simulink model "downlink_4c2t"  (Simulink 8.7)
settings: Solver=VariableStepDiscrete  StartTime=0.0  StopTime=DUC_LINEUP_param.endTime  RelTol=1e-3
PreLoadFcn:
  | % Run the setup script when the model is opened
  | setup_downlink_4c2t;
InitFcn:
  | % Run the setup script again just before the
  | % model is run, so that any updates made
  | % after opening are applied.
  | setup_downlink_4c2t;
  | 
  | %% DSPBuilder Start
  | alt_dspbuilder_update_model(bdroot)
  | %% DSPBuilder End
values from neighbouring files (symbols this model uses):
  LUTS_DPD_CLIP =     [downlink_4c2t_dpd_clip.mat]
  PulsExtention = 128    [setup_downlink_4c2t.m]
  StartAddress1 = Iter1_Param.BaseAddr + 3200    [setup_downlink_4c2t.m]
  StartAddress2 = StartAddress1+1024    [setup_downlink_4c2t.m]
  win = [w(1:PulsExtention) ones(1,Iter0_Param.pulseLen) w(PulsExtention+1:end)]    [setup_downlink_4c2t.m]
undefined symbols (not defined in the file or in its folder): AdvDSPBChannelOutDisplay, AdvDSPBDMemDisplay, dpoly, dspba_ChannelInVis, dspba_ChannelOutVis, dspba_internal_get_channel_ports, dspba_internal_get_demux_ports, DUC_LINEUP_param, evalAionMaskParam, iq_width, Iter0_Param, latency, primtype, REG, UseDontCare, value
undefined symbols (not defined in the file): cfr0_id, cfr_Params0, cfr_Params1, clock_rate, REG_dut_id_addr
libraries: DSPBAPrim x1438, DSPBAControl x77, DSPBAModelBus x71, DSPBABase x40, downlink_4c2t_foldingcfr_3firs_lib x26, DSPBAUtilities x8, downlink_4c2t_lib x4, downlink_4c2t_cordic_lib x2, downlink_4c2t_dpd_clipper x2, DSPBAFilters x2, DSPBAWaveformSynth x2, downlink_4c2t_lduc_lib x1
(part 3 of 17)

== system downlink_4c2t/DUT/Gain_duc_input ==
  a : Inport
  v : Inport  Port=2
  c : Inport  Port=3
  carr1_gain_val : Inport  Port=4
  carr2_gain_val : Inport  Port=5
  carr3_gain_val : Inport  Port=6
  carr4_gain_val : Inport  Port=7
  carr5_gain_val : Inport  Port=8
  carr6_gain_val : Inport  Port=9
  carr7_gain_val : Inport  Port=10
  carr8_gain_val : Inport  Port=11
  Term : Terminator
  gain : Subsystem
  scale_gain : DSPBABase/Scale  otype=sfix(16 )  scale=2^-15  rndmethod=Unbiased  factor=1  satmethod=Symmetric  shift_vec=0  latency=7  wideSimulation=off  version=20090407
  zero_idx : DSPBAPrim/Const  primtype=const  nInputs=0  nOutputs=1  omode=Inherit via internal rule  otype=sfix(16)  scale=2^-15  rndmethod=Unbiased  factor=1  satmethod=Symmetric  shift_vec=[0 1 2 -1]  value=0  inPortNames=['+'; '+';]  outPortNames=[' ']  dspbaimage=dspba_prim.jpg  text=fprintf('%s', num2str(value));  style=Optimised  visibilities=8 + 1024  floatPrecision=float32_m23  version=20120820
  gain_v_out : Outport
  gain_c_out : Outport  Port=2
  gain_real_out : Outport  Port=3
  wires:
  a/1 -> gain/1(a)
  v/1 -> gain/2(v)
  c/1 -> gain/3(c)
  scale_gain/4 -> Term/1
  zero_idx/1 -> scale_gain/4
  gain/1(gain_v_out) -> scale_gain/2
  gain/2(gain_c_out) -> scale_gain/3
  gain/3(gain_real_out) -> scale_gain/1
  scale_gain/1 -> gain_real_out/1
  scale_gain/2 -> gain_v_out/1
  scale_gain/3 -> gain_c_out/1
  carr1_gain_val/1 -> gain/4(carr1_gain_val)
  carr2_gain_val/1 -> gain/5(carr2_gain_val)
  carr3_gain_val/1 -> gain/6(carr3_gain_val)
  carr4_gain_val/1 -> gain/7(carr4_gain_val)
  carr5_gain_val/1 -> gain/8(carr5_gain_val)
  carr6_gain_val/1 -> gain/9(carr6_gain_val)
  carr7_gain_val/1 -> gain/10(carr7_gain_val)
  carr8_gain_val/1 -> gain/11(carr8_gain_val)

== system downlink_4c2t/DUT/Gain_summer ==
  a : Inport
  v : Inport  Port=2
  c : Inport  Port=3
  Ant1_gain_val : Inport  Port=4
  Antr2_gain_val : Inport  Port=5
  Subsystem : Subsystem
  Term : Terminator
  scale_gain : DSPBABase/Scale  otype=sfix(16 )  scale=2^-15  rndmethod=Unbiased  factor=1  satmethod=Symmetric  shift_vec=0  latency=7  wideSimulation=off  version=20090407
  zero_idx : DSPBAPrim/Const  primtype=const  nInputs=0  nOutputs=1  omode=Inherit via internal rule  otype=sfix(16)  scale=2^-15  rndmethod=Unbiased  factor=1  satmethod=Symmetric  shift_vec=[0 1 2 -1]  value=0  inPortNames=['+'; '+';]  outPortNames=[' ']  dspbaimage=dspba_prim.jpg  text=fprintf('%s', num2str(value));  style=Optimised  visibilities=8 + 1024  floatPrecision=float32_m23  version=20120820
  gain_real_out : Outport
  gain_v_out : Outport  Port=2
  gain_c_out : Outport  Port=3
  wires:
  Antr2_gain_val/1 -> Subsystem/5(ant2_gain_val)
  Ant1_gain_val/1 -> Subsystem/4(ant1_gain_val)
  scale_gain/3 -> gain_c_out/1
  scale_gain/2 -> gain_v_out/1
  scale_gain/1 -> gain_real_out/1
  Subsystem/3(gain_real_out) -> scale_gain/1
  Subsystem/2(gain_c_out) -> scale_gain/3
  Subsystem/1(gain_v_out) -> scale_gain/2
  zero_idx/1 -> scale_gain/4
  scale_gain/4 -> Term/1
  c/1 -> Subsystem/3(c)
  v/1 -> Subsystem/2(v)
  a/1 -> Subsystem/1(a)

== system downlink_4c2t/DUT/HDUC_STG1 ==
  a1 : Inport
  v : Inport  Port=2
  c : Inport  Port=3
  Const5 : DSPBAPrim/Const  primtype=const  nInputs=0  nOutputs=1  omode=Inherit via internal rule  otype=sfix(16)  scale=2^-15  rndmethod=Unbiased  factor=1  satmethod=Symmetric  shift_vec=[0 1 2 -1]  value=0  inPortNames=['+'; '+';]  outPortNames=[' ']  dspbaimage=dspba_prim.jpg  text=fprintf('%s', num2str(value));  style=Optimised  visibilities=8 + 1024  floatPrecision=float32_m23  version=20120820
  HB_filter6 : DSPBAFilters/InterpolatingFIR  nInputRate=DUC_LINEUP_param.HB_filt6.SampleRate  interp=DUC_LINEUP_param.HB_filt6.Interpolation  nchan=DUC_LINEUP_param.HB_filt6.ChanCount  symmetry=Symmetrical  coef=DUC_LINEUP_param.HB_filt6.coeffs(1,:)  addr=DUC_LINEUP_param.HB_filt6.base_addr1  rwmode=Read/Write  nband=Half Band  exposebus=off  latency=9  version=20090407  recon=off  MM=[0,1,2,3,4,5,6,7,8,9,10,11,12,13,14,15]
  Terminator : Terminator
  scale_HB_filter6 : DSPBABase/Scale  otype=sfix(DUC_LINEUP_param.output_word_length)  scale=2^-DUC_LINEUP_param.output_fraction_length  rndmethod=Truncate  factor=[1 1]  satmethod=Symmetric  shift_vec=[1 1]  latency=7  wideSimulation=off  version=20090407
  q1 : Outport
  qv : Outport  Port=2
  qc : Outport  Port=3
  wires:
  scale_HB_filter6/1 -> q1/1
  scale_HB_filter6/3 -> qc/1
  HB_filter6/3 -> scale_HB_filter6/3
  HB_filter6/2 -> scale_HB_filter6/2
  scale_HB_filter6/2 -> qv/1
  HB_filter6/1 -> scale_HB_filter6/1
  Const5/1 -> scale_HB_filter6/4
  v/1 -> HB_filter6/2
  c/1 -> HB_filter6/3
  a1/1 -> HB_filter6/1
  scale_HB_filter6/4 -> Terminator/1

== system downlink_4c2t/DUT/HDUC_STG2 ==
  a1 : Inport
  v : Inport  Port=2
  c : Inport  Port=3
  Const5 : DSPBAPrim/Const  primtype=const  nInputs=0  nOutputs=1  omode=Specify via dialog  otype=ufix(2)  scale=2^-0  rndmethod=Unbiased  factor=1  satmethod=Symmetric  shift_vec=[0 1 2 -1]  value=0  inPortNames=['+'; '+';]  outPortNames=[' ']  dspbaimage=dspba_prim.jpg  text=fprintf('%s', num2str(value));  style=Optimised  visibilities=8 + 1024  floatPrecision=float32_m23  version=20120820
  HB_filter7 : DSPBAFilters/InterpolatingFIR  nInputRate=DUC_LINEUP_param.HB_filt7.SampleRate  interp=DUC_LINEUP_param.HB_filt7.Interpolation  nchan=DUC_LINEUP_param.HB_filt7.ChanCount  symmetry=Symmetrical  coef=DUC_LINEUP_param.HB_filt7.coeffs(1,:)  addr=DUC_LINEUP_param.HB_filt7.base_addr1  rwmode=Read/Write  nband=Half Band  exposebus=off  latency=7  version=20090407  recon=off  MM=[0,1,2,3,4,5,6,7,8,9,10,11,12,13,14,15]
  Terminator : Terminator
  scale_HB_filter6 : DSPBABase/Scale  otype=sfix(DUC_LINEUP_param.output_word_length)  scale=2^-DUC_LINEUP_param.output_fraction_length  rndmethod=Truncate  factor=[1 1 1 1]  satmethod=Symmetric  shift_vec=[1 1 1 1]  latency=7  wideSimulation=off  version=20090407
  q1 : Outport
  qv : Outport  Port=2
  qc : Outport  Port=3
  wires:
  scale_HB_filter6/1 -> q1/1
  scale_HB_filter6/3 -> qc/1
  HB_filter7/3 -> scale_HB_filter6/3
  HB_filter7/2 -> scale_HB_filter6/2
  scale_HB_filter6/2 -> qv/1
  HB_filter7/1 -> scale_HB_filter6/1
  Const5/1 -> scale_HB_filter6/4
  v/1 -> HB_filter7/2
  c/1 -> HB_filter7/3
  a1/1 -> HB_filter7/1
  scale_HB_filter6/4 -> Terminator/1

== system downlink_4c2t/DUT/LDUC ==
  In_v : Inport
  In_c : Inport  Port=2
  In_d : Inport  Port=3
  In_sync_pulse : Inport  Port=4
  sum_shift : Inport  Port=5
  LDUC : downlink_4c2t_lduc_lib/LDUC1  clock_margin=DUC_LINEUP_param.ClockMargin_DUC  chan_filter_base_addr=DUC_LINEUP_param.chan_filter.base_addr1  hb4_base_addr=DUC_LINEUP_param.HB_filt4.base_addr1  hb5_base_addr=DUC_LINEUP_param.HB_filt5.base_addr1  hb5_2_base_addr=DUC_LINEUP_param.HB_filt5_2.base_addr1
      link override Channal_Filter/SingleRateFIR: latency=4
      link override Channal_Filter/scale_HB_filter1: latency=4
      link override HB4/HB4/HB_filter4: latency=15
      link override HB4/HB4/scale_HB_filter4: latency=4
      link override HB5/HB_filter5: latency=11
      link override HB5/HB_filter_2: latency=11
      link override HB5/PipeReg1/ChannelOut: value=1  packetBeginEnabled=off  latency=1
      link override HB5/PipeReg2/ChannelOut: value=1  packetBeginEnabled=off  latency=1
      link override HB5/PipeReg3/ChannelOut: value=1  packetBeginEnabled=off  latency=1
      link override HB5/PipeReg4/ChannelOut: value=1  packetBeginEnabled=off  latency=1
      link override HB5/scale_HB_filter5: latency=4
      link override PipeReg/ChannelOut: value=1  packetBeginEnabled=off  latency=2
      link override PipeReg1/ChannelOut: value=1  packetBeginEnabled=off  latency=1
      link override PipeReg2/ChannelOut: value=1  packetBeginEnabled=off  latency=2
      link override PipeReg3/ChannelOut: value=1  packetBeginEnabled=off  latency=1
      link override PipeReg4/ChannelOut: value=1  packetBeginEnabled=off  latency=2
      link override PipeReg5/ChannelOut: value=1  packetBeginEnabled=off  latency=2
  Mixer_Summer : Subsystem
  PipeReg_avln_lduc_L : downlink_4c2t_foldingcfr_3firs_lib/PipeReg  NPipe=2  Clock_Margin=DUC_LINEUP_param.ClockMargin
      link override ChannelOut: latency=2  value=1  packetBeginEnabled=off
  PipeReg_avln_lduc_R : downlink_4c2t_foldingcfr_3firs_lib/PipeReg  NPipe=2  Clock_Margin=DUC_LINEUP_param.ClockMargin
      link override ChannelOut: latency=2  value=1  packetBeginEnabled=off
  Out1 : Outport
  Out2 : Outport  Port=2
  Out3 : Outport  Port=3
  wires:
  PipeReg_avln_lduc_R/1 -> LDUC/1
  PipeReg_avln_lduc_R/2 -> LDUC/2
  In_v/1 -> PipeReg_avln_lduc_L/2
  In_d/1 -> PipeReg_avln_lduc_L/1
  PipeReg_avln_lduc_L/2 -> PipeReg_avln_lduc_R/2
  PipeReg_avln_lduc_L/3 -> PipeReg_avln_lduc_R/3
  In_c/1 -> PipeReg_avln_lduc_L/3
  PipeReg_avln_lduc_R/3 -> LDUC/3
  In_sync_pulse/1 -> Mixer_Summer/4(In_sync_pulse)
  LDUC/1 -> Mixer_Summer/1(In_a)
  LDUC/2 -> Mixer_Summer/2(In_V)
  LDUC/3 -> Mixer_Summer/3(In_C)
  Mixer_Summer/3(Out_C) -> Out3/1
  Mixer_Summer/1(Out_q) -> Out1/1
  Mixer_Summer/2(Out_V) -> Out2/1
  PipeReg_avln_lduc_L/1 -> PipeReg_avln_lduc_R/1
  sum_shift/1 -> Mixer_Summer/5(sum_shift)

== system downlink_4c2t/DUT/REAL_COMPLEX1 ==
  a1 : Inport
  v : Inport  Port=2
  c : Inport  Port=3
  ChannelIn : DSPBAPrim/ChannelIn  primtype=channelin  nInputs=dspba_internal_get_channel_ports(gcb)  nOutputs=dspba_internal_get_channel_ports(gcb)  omode=Inherit via internal rule  otype=sfix(16)  scale=2^-15  rndmethod=Unbiased  factor=1  satmethod=Symmetric  shift_vec=[0 1 2 -1]  value=1  inPortNames=['v'; 'c'; '0'; '1'; '2'; '3'; '4'; '5'; '6'; '7'; '8'; '9'; 'A'; 'B'; 'D'; 'E'; 'F'; 'G'; 'H'; 'I'; 'J'; 'K'; 'L'; 'M'; 'N'; 'O'; 'P'; 'Q'; 'R'; 'S'; 'T'; 'U'; 'W'; 'X'; 'Y'; 'Z']  outPortNames=['v'; 'c'; '0'; '1'; '2'; '3'; '4'; '5'; '6'; '7'; '8'; '9'; 'A'; 'B'; 'D'; 'E'; 'F'; 'G'; 'H'; 'I'; 'J'; 'K'; 'L'; 'M'; 'N'; 'O'; 'P'; 'Q'; 'R'; 'S'; 'T'; 'U'; 'W'; 'X'; 'Y'; 'Z']  dspbaimage=dspba_prim.jpg  text=fprintf('In');  style=Optimised  dataSignals=1  foldingEnabled=off  channels=1  sampleRate=200  packetBeginPresent=off  packetBeginEnabled=off  visibilities=dspba_ChannelInVis(gcb)  latencyCorrection=0  version=20141013
  ChannelOut : DSPBAPrim/ChannelOut  primtype=channelout  nInputs=dspba_internal_get_channel_ports(gcb)  nOutputs=dspba_internal_get_channel_ports(gcb)  omode=Inherit via internal rule  otype=sfix(16)  scale=2^-15  rndmethod=Unbiased  factor=1  satmethod=Symmetric  shift_vec=[0 1 2 -1]  value=4  inPortNames=['v'; 'c'; '0'; '1'; '2'; '3'; '4'; '5'; '6'; '7'; '8'; '9'; 'A'; 'B'; 'D'; 'E'; 'F'; 'G'; 'H'; 'I'; 'J'; 'K'; 'L'; 'M'; 'N'; 'O'; 'P'; 'Q'; 'R'; 'S'; 'T'; 'U'; 'W'; 'X'; 'Y'; 'Z']  outPortNames=['v'; 'c'; '0'; '1'; '2'; '3'; '4'; '5'; '6'; '7'; '8'; '9'; 'A'; 'B'; 'D'; 'E'; 'F'; 'G'; 'H'; 'I'; 'J'; 'K'; 'L'; 'M'; 'N'; 'O'; 'P'; 'Q'; 'R'; 'S'; 'T'; 'U'; 'W'; 'X'; 'Y'; 'Z']  dspbaimage=dspba_prim.jpg  text=fprintf('Out%s', AdvDSPBChannelOutDisplay(latency));  style=Optimised  dataSignals=4  foldingEnabled=off  channels=1  sampleRate=200  packetBeginPresent=off  packetBeginEnabled=off  visibilities=dspba_ChannelOutVis(gcb)  latency=0  latencyCorrection=0  version=20141013
  Const : DSPBAPrim/Const  primtype=const  nInputs=0  nOutputs=1  omode=Inherit via internal rule  otype=sfix(16)  scale=2^-15  rndmethod=Unbiased  factor=1  satmethod=Symmetric  shift_vec=[0 1 2 -1]  value=0  inPortNames=['+'; '+';]  outPortNames=[' ']  dspbaimage=dspba_prim.jpg  text=fprintf('%s', num2str(value));  style=Optimised  visibilities=8 + 1024  floatPrecision=float32_m23  version=20120820
  Demux4 : Demux
  LocalThreshold : DSPBABase/LocalThreshold  margin=DUC_LINEUP_param.ClockMargin  delayRegOrRAMThresholdBits=-1  MediumDualMemThresholdBits=-1  LargeDualMemThresholdBits=-1  hardMultiplierThresholdLuts=-1  complexMultKaratsuba=off  version=0
  Real-Imag to Complex : RealImagToComplex
  Real-Imag to Complex1 : RealImagToComplex
  SynthesisInfo : DSPBAPrim/SynthesisInfo  primtype=synthinfo  nInputs=0  nOutputs=0  omode=Inherit via internal rule  otype=sfix(16)  scale=2^-15  rndmethod=Truncate  factor=1  satmethod=Symmetric  shift_vec=[0 1 2 -1]  value=99  inPortNames=[' '; ' ';]  outPortNames=[' ']  dspbaimage=dspba_prim_ctrl.jpg  text=fprintf('Style=%s', style);  style=Scheduled  visibilities=2^15+2^17+2^18+2^19  constraintInUse=off  constraintRelation=>  constraintLimit=20  bitAccurate=off  version=20150220
  Terminator17 : Terminator
  q1 : Outport
  q2 : Outport  Port=2
  q_v : Outport  Port=3
  q_c : Outport  Port=4
  wires:
  ChannelOut/3 -> Real-Imag to Complex/1
  Demux4/2 -> ChannelOut/4
  Demux4/4 -> ChannelOut/6
  Demux4/3 -> ChannelOut/5
  ChannelIn/2 -> Terminator17/1
  Const/1 -> ChannelOut/2
  ChannelIn/1 -> ChannelOut/1
  Demux4/1 -> ChannelOut/3
  ChannelIn/3 -> Demux4/1
  Real-Imag to Complex/1 -> q1/1
  ChannelOut/4 -> Real-Imag to Complex/2
  ChannelOut/2 -> q_c/1
  ChannelOut/1 -> q_v/1
  c/1 -> ChannelIn/2
  v/1 -> ChannelIn/1
  a1/1 -> ChannelIn/3
  Real-Imag to Complex1/1 -> q2/1
  ChannelOut/5 -> Real-Imag to Complex1/1
  ChannelOut/6 -> Real-Imag to Complex1/2

== system downlink_4c2t/DUT/REAL_COMPLEX2 ==
  a1 : Inport
  v : Inport  Port=2
  c : Inport  Port=3
  ChannelIn : DSPBAPrim/ChannelIn  primtype=channelin  nInputs=dspba_internal_get_channel_ports(gcb)  nOutputs=dspba_internal_get_channel_ports(gcb)  omode=Inherit via internal rule  otype=sfix(16)  scale=2^-15  rndmethod=Unbiased  factor=1  satmethod=Symmetric  shift_vec=[0 1 2 -1]  value=1  inPortNames=['v'; 'c'; '0'; '1'; '2'; '3'; '4'; '5'; '6'; '7'; '8'; '9'; 'A'; 'B'; 'D'; 'E'; 'F'; 'G'; 'H'; 'I'; 'J'; 'K'; 'L'; 'M'; 'N'; 'O'; 'P'; 'Q'; 'R'; 'S'; 'T'; 'U'; 'W'; 'X'; 'Y'; 'Z']  outPortNames=['v'; 'c'; '0'; '1'; '2'; '3'; '4'; '5'; '6'; '7'; '8'; '9'; 'A'; 'B'; 'D'; 'E'; 'F'; 'G'; 'H'; 'I'; 'J'; 'K'; 'L'; 'M'; 'N'; 'O'; 'P'; 'Q'; 'R'; 'S'; 'T'; 'U'; 'W'; 'X'; 'Y'; 'Z']  dspbaimage=dspba_prim.jpg  text=fprintf('In');  style=Optimised  dataSignals=1  foldingEnabled=off  channels=1  sampleRate=200  packetBeginPresent=off  packetBeginEnabled=off  visibilities=dspba_ChannelInVis(gcb)  latencyCorrection=0  version=20141013
  ChannelOut : DSPBAPrim/ChannelOut  primtype=channelout  nInputs=dspba_internal_get_channel_ports(gcb)  nOutputs=dspba_internal_get_channel_ports(gcb)  omode=Inherit via internal rule  otype=sfix(16)  scale=2^-15  rndmethod=Unbiased  factor=1  satmethod=Symmetric  shift_vec=[0 1 2 -1]  value=4  inPortNames=['v'; 'c'; '0'; '1'; '2'; '3'; '4'; '5'; '6'; '7'; '8'; '9'; 'A'; 'B'; 'D'; 'E'; 'F'; 'G'; 'H'; 'I'; 'J'; 'K'; 'L'; 'M'; 'N'; 'O'; 'P'; 'Q'; 'R'; 'S'; 'T'; 'U'; 'W'; 'X'; 'Y'; 'Z']  outPortNames=['v'; 'c'; '0'; '1'; '2'; '3'; '4'; '5'; '6'; '7'; '8'; '9'; 'A'; 'B'; 'D'; 'E'; 'F'; 'G'; 'H'; 'I'; 'J'; 'K'; 'L'; 'M'; 'N'; 'O'; 'P'; 'Q'; 'R'; 'S'; 'T'; 'U'; 'W'; 'X'; 'Y'; 'Z']  dspbaimage=dspba_prim.jpg  text=fprintf('Out%s', AdvDSPBChannelOutDisplay(latency));  style=Optimised  dataSignals=4  foldingEnabled=off  channels=1  sampleRate=200  packetBeginPresent=off  packetBeginEnabled=off  visibilities=dspba_ChannelOutVis(gcb)  latency=0  latencyCorrection=0  version=20141013
  Const : DSPBAPrim/Const  primtype=const  nInputs=0  nOutputs=1  omode=Inherit via internal rule  otype=sfix(16)  scale=2^-15  rndmethod=Unbiased  factor=1  satmethod=Symmetric  shift_vec=[0 1 2 -1]  value=0  inPortNames=['+'; '+';]  outPortNames=[' ']  dspbaimage=dspba_prim.jpg  text=fprintf('%s', num2str(value));  style=Optimised  visibilities=8 + 1024  floatPrecision=float32_m23  version=20120820
  Demux4 : Demux
  LocalThreshold : DSPBABase/LocalThreshold  margin=DUC_LINEUP_param.ClockMargin  delayRegOrRAMThresholdBits=-1  MediumDualMemThresholdBits=-1  LargeDualMemThresholdBits=-1  hardMultiplierThresholdLuts=-1  complexMultKaratsuba=off  version=0
  Real-Imag to Complex : RealImagToComplex
  Real-Imag to Complex1 : RealImagToComplex
  SynthesisInfo : DSPBAPrim/SynthesisInfo  primtype=synthinfo  nInputs=0  nOutputs=0  omode=Inherit via internal rule  otype=sfix(16)  scale=2^-15  rndmethod=Truncate  factor=1  satmethod=Symmetric  shift_vec=[0 1 2 -1]  value=99  inPortNames=[' '; ' ';]  outPortNames=[' ']  dspbaimage=dspba_prim_ctrl.jpg  text=fprintf('Style=%s', style);  style=Scheduled  visibilities=2^15+2^17+2^18+2^19  constraintInUse=off  constraintRelation=>  constraintLimit=20  bitAccurate=off  version=20150220
  Terminator17 : Terminator
  q1 : Outport
  q2 : Outport  Port=2
  q_v : Outport  Port=3
  q_c : Outport  Port=4
  wires:
  ChannelOut/6 -> Real-Imag to Complex1/2
  ChannelOut/5 -> Real-Imag to Complex1/1
  Real-Imag to Complex1/1 -> q2/1
  a1/1 -> ChannelIn/3
  v/1 -> ChannelIn/1
  c/1 -> ChannelIn/2
  ChannelOut/1 -> q_v/1
  ChannelOut/2 -> q_c/1
  ChannelOut/4 -> Real-Imag to Complex/2
  Real-Imag to Complex/1 -> q1/1
  ChannelIn/3 -> Demux4/1
  Demux4/1 -> ChannelOut/3
  ChannelIn/1 -> ChannelOut/1
  Const/1 -> ChannelOut/2
  ChannelIn/2 -> Terminator17/1
  Demux4/3 -> ChannelOut/5
  Demux4/4 -> ChannelOut/6
  Demux4/2 -> ChannelOut/4
  ChannelOut/3 -> Real-Imag to Complex/1

== system downlink_4c2t/DUT/dpd_ant1_out_rfp ==
  GPOut : DSPBAPrim/GPOut  primtype=gpout  nInputs=evalAionMaskParam(gcb,'value',1)  nOutputs=evalAionMaskParam(gcb,'value',1)  omode=Inherit via internal rule  otype=sfix(16)  scale=2^-15  rndmethod=Unbiased  factor=1  satmethod=Symmetric  shift_vec=[0 1 2 -1]  value=1  inPortNames=[' ' ' ' ' ' ' ' ' ' ' ' ' ' ' ' ' ' ' ' ' ' ' ' ' ' ' ' ' ' ' ' ' ' ' ' ' ' ' ' ' ' ' ' ' ' ' ' ' ' ' ' ' ' ' ' ' ' ' ' ' ' ' ' ' ' ' ' ' ']'  outPortNames=[' ' ' ' ' ' ' ' ' ' ' ' ' ' ' ' ' ' ' ' ' ' ' ' ' ' ' ' ' ' ' ' ' ' ' ' ' ' ' ' ' ' ' ' ' ' ' ' ' ' ' ' ' ' ' ' ' ' ' ' ' ' ' ' ' ' ' ' ' ']'  dspbaimage=dspba_prim.jpg  text=fprintf('GPOut');  style=Optimised  visibilities=1024  latencyCorrection=0  version=20090407
  SynthesisInfo : DSPBAPrim/SynthesisInfo  primtype=synthinfo  nInputs=0  nOutputs=0  omode=Inherit via internal rule  otype=sfix(16)  scale=2^-15  rndmethod=Truncate  factor=1  satmethod=Symmetric  shift_vec=[0 1 2 -1]  value=99  inPortNames=[' '; ' ';]  outPortNames=[' ']  dspbaimage=dspba_prim_ctrl.jpg  text=fprintf('Style=%s', style);  style=Scheduled  visibilities=2^15+2^17+2^18+2^19  constraintInUse=off  constraintRelation=>  constraintLimit=2  bitAccurate=off  version=20150220
  zero_idx1 : DSPBAPrim/Const  primtype=const  nInputs=0  nOutputs=1  omode=boolean  otype=ufix(1)  scale=0  rndmethod=Unbiased  factor=1  satmethod=Symmetric  shift_vec=[0 1 2 -1]  value=1  inPortNames=['+'; '+';]  outPortNames=[' ']  dspbaimage=dspba_prim.jpg  text=fprintf('%s', num2str(value));  style=Optimised  visibilities=8 + 1024  floatPrecision=float32_m23  version=20120820
  Out_RFP : Outport
  wires:
  GPOut/1 -> Out_RFP/1
  zero_idx1/1 -> GPOut/1

== system downlink_4c2t/DUT/dpd_ant2_out_rfp ==
  GPOut : DSPBAPrim/GPOut  primtype=gpout  nInputs=evalAionMaskParam(gcb,'value',1)  nOutputs=evalAionMaskParam(gcb,'value',1)  omode=Inherit via internal rule  otype=sfix(16)  scale=2^-15  rndmethod=Unbiased  factor=1  satmethod=Symmetric  shift_vec=[0 1 2 -1]  value=1  inPortNames=[' ' ' ' ' ' ' ' ' ' ' ' ' ' ' ' ' ' ' ' ' ' ' ' ' ' ' ' ' ' ' ' ' ' ' ' ' ' ' ' ' ' ' ' ' ' ' ' ' ' ' ' ' ' ' ' ' ' ' ' ' ' ' ' ' ' ' ' ' ']'  outPortNames=[' ' ' ' ' ' ' ' ' ' ' ' ' ' ' ' ' ' ' ' ' ' ' ' ' ' ' ' ' ' ' ' ' ' ' ' ' ' ' ' ' ' ' ' ' ' ' ' ' ' ' ' ' ' ' ' ' ' ' ' ' ' ' ' ' ' ' ' ' ']'  dspbaimage=dspba_prim.jpg  text=fprintf('GPOut');  style=Optimised  visibilities=1024  latencyCorrection=0  version=20090407
  SynthesisInfo : DSPBAPrim/SynthesisInfo  primtype=synthinfo  nInputs=0  nOutputs=0  omode=Inherit via internal rule  otype=sfix(16)  scale=2^-15  rndmethod=Truncate  factor=1  satmethod=Symmetric  shift_vec=[0 1 2 -1]  value=99  inPortNames=[' '; ' ';]  outPortNames=[' ']  dspbaimage=dspba_prim_ctrl.jpg  text=fprintf('Style=%s', style);  style=Scheduled  visibilities=2^15+2^17+2^18+2^19  constraintInUse=off  constraintRelation=>  constraintLimit=2  bitAccurate=off  version=20150220
  zero_idx1 : DSPBAPrim/Const  primtype=const  nInputs=0  nOutputs=1  omode=boolean  otype=ufix(1)  scale=0  rndmethod=Unbiased  factor=1  satmethod=Symmetric  shift_vec=[0 1 2 -1]  value=1  inPortNames=['+'; '+';]  outPortNames=[' ']  dspbaimage=dspba_prim.jpg  text=fprintf('%s', num2str(value));  style=Optimised  visibilities=8 + 1024  floatPrecision=float32_m23  version=20120820
  Out_RFP : Outport
  wires:
  zero_idx1/1 -> GPOut/1
  GPOut/1 -> Out_RFP/1

== system downlink_4c2t/DUT/lcfr_rfp ==
  GPOut : DSPBAPrim/GPOut  primtype=gpout  nInputs=evalAionMaskParam(gcb,'value',1)  nOutputs=evalAionMaskParam(gcb,'value',1)  omode=Inherit via internal rule  otype=sfix(16)  scale=2^-15  rndmethod=Unbiased  factor=1  satmethod=Symmetric  shift_vec=[0 1 2 -1]  value=1  inPortNames=[' ' ' ' ' ' ' ' ' ' ' ' ' ' ' ' ' ' ' ' ' ' ' ' ' ' ' ' ' ' ' ' ' ' ' ' ' ' ' ' ' ' ' ' ' ' ' ' ' ' ' ' ' ' ' ' ' ' ' ' ' ' ' ' ' ' ' ' ' ']'  outPortNames=[' ' ' ' ' ' ' ' ' ' ' ' ' ' ' ' ' ' ' ' ' ' ' ' ' ' ' ' ' ' ' ' ' ' ' ' ' ' ' ' ' ' ' ' ' ' ' ' ' ' ' ' ' ' ' ' ' ' ' ' ' ' ' ' ' ' ' ' ' ']'  dspbaimage=dspba_prim.jpg  text=fprintf('GPOut');  style=Optimised  visibilities=1024  latencyCorrection=0  version=20090407
  SynthesisInfo : DSPBAPrim/SynthesisInfo  primtype=synthinfo  nInputs=0  nOutputs=0  omode=Inherit via internal rule  otype=sfix(16)  scale=2^-15  rndmethod=Truncate  factor=1  satmethod=Symmetric  shift_vec=[0 1 2 -1]  value=99  inPortNames=[' '; ' ';]  outPortNames=[' ']  dspbaimage=dspba_prim_ctrl.jpg  text=fprintf('Style=%s', style);  style=Scheduled  visibilities=2^15+2^17+2^18+2^19  constraintInUse=off  constraintRelation=>  constraintLimit=2  bitAccurate=off  version=20150220
  zero_idx1 : DSPBAPrim/Const  primtype=const  nInputs=0  nOutputs=1  omode=boolean  otype=ufix(1)  scale=0  rndmethod=Unbiased  factor=1  satmethod=Symmetric  shift_vec=[0 1 2 -1]  value=1  inPortNames=['+'; '+';]  outPortNames=[' ']  dspbaimage=dspba_prim.jpg  text=fprintf('%s', num2str(value));  style=Optimised  visibilities=8 + 1024  floatPrecision=float32_m23  version=20120820
  Out_RFP : Outport
  wires:
  GPOut/1 -> Out_RFP/1
  zero_idx1/1 -> GPOut/1

== system downlink_4c2t/DUT/lcfr_rfp1 ==
  GPOut : DSPBAPrim/GPOut  primtype=gpout  nInputs=evalAionMaskParam(gcb,'value',1)  nOutputs=evalAionMaskParam(gcb,'value',1)  omode=Inherit via internal rule  otype=sfix(16)  scale=2^-15  rndmethod=Unbiased  factor=1  satmethod=Symmetric  shift_vec=[0 1 2 -1]  value=1  inPortNames=[' ' ' ' ' ' ' ' ' ' ' ' ' ' ' ' ' ' ' ' ' ' ' ' ' ' ' ' ' ' ' ' ' ' ' ' ' ' ' ' ' ' ' ' ' ' ' ' ' ' ' ' ' ' ' ' ' ' ' ' ' ' ' ' ' ' ' ' ' ']'  outPortNames=[' ' ' ' ' ' ' ' ' ' ' ' ' ' ' ' ' ' ' ' ' ' ' ' ' ' ' ' ' ' ' ' ' ' ' ' ' ' ' ' ' ' ' ' ' ' ' ' ' ' ' ' ' ' ' ' ' ' ' ' ' ' ' ' ' ' ' ' ' ']'  dspbaimage=dspba_prim.jpg  text=fprintf('GPOut');  style=Optimised  visibilities=1024  latencyCorrection=0  version=20090407
  SynthesisInfo : DSPBAPrim/SynthesisInfo  primtype=synthinfo  nInputs=0  nOutputs=0  omode=Inherit via internal rule  otype=sfix(16)  scale=2^-15  rndmethod=Truncate  factor=1  satmethod=Symmetric  shift_vec=[0 1 2 -1]  value=99  inPortNames=[' '; ' ';]  outPortNames=[' ']  dspbaimage=dspba_prim_ctrl.jpg  text=fprintf('Style=%s', style);  style=Scheduled  visibilities=2^15+2^17+2^18+2^19  constraintInUse=off  constraintRelation=>  constraintLimit=2  bitAccurate=off  version=20150220
  zero_idx1 : DSPBAPrim/Const  primtype=const  nInputs=0  nOutputs=1  omode=boolean  otype=ufix(1)  scale=0  rndmethod=Unbiased  factor=1  satmethod=Symmetric  shift_vec=[0 1 2 -1]  value=1  inPortNames=['+'; '+';]  outPortNames=[' ']  dspbaimage=dspba_prim.jpg  text=fprintf('%s', num2str(value));  style=Optimised  visibilities=8 + 1024  floatPrecision=float32_m23  version=20120820
  Out_RFP : Outport
  wires:
  zero_idx1/1 -> GPOut/1
  GPOut/1 -> Out_RFP/1

== system downlink_4c2t/DUT/lduc_bypass_rfp ==
  GPOut : DSPBAPrim/GPOut  primtype=gpout  nInputs=evalAionMaskParam(gcb,'value',1)  nOutputs=evalAionMaskParam(gcb,'value',1)  omode=Inherit via internal rule  otype=sfix(16)  scale=2^-15  rndmethod=Unbiased  factor=1  satmethod=Symmetric  shift_vec=[0 1 2 -1]  value=1  inPortNames=[' ' ' ' ' ' ' ' ' ' ' ' ' ' ' ' ' ' ' ' ' ' ' ' ' ' ' ' ' ' ' ' ' ' ' ' ' ' ' ' ' ' ' ' ' ' ' ' ' ' ' ' ' ' ' ' ' ' ' ' ' ' ' ' ' ' ' ' ' ']'  outPortNames=[' ' ' ' ' ' ' ' ' ' ' ' ' ' ' ' ' ' ' ' ' ' ' ' ' ' ' ' ' ' ' ' ' ' ' ' ' ' ' ' ' ' ' ' ' ' ' ' ' ' ' ' ' ' ' ' ' ' ' ' ' ' ' ' ' ' ' ' ' ']'  dspbaimage=dspba_prim.jpg  text=fprintf('GPOut');  style=Optimised  visibilities=1024  latencyCorrection=0  version=20090407
  SynthesisInfo : DSPBAPrim/SynthesisInfo  primtype=synthinfo  nInputs=0  nOutputs=0  omode=Inherit via internal rule  otype=sfix(16)  scale=2^-15  rndmethod=Truncate  factor=1  satmethod=Symmetric  shift_vec=[0 1 2 -1]  value=99  inPortNames=[' '; ' ';]  outPortNames=[' ']  dspbaimage=dspba_prim_ctrl.jpg  text=fprintf('Style=%s', style);  style=Scheduled  visibilities=2^15+2^17+2^18+2^19  constraintInUse=off  constraintRelation=>  constraintLimit=2  bitAccurate=off  version=20150220
  zero_idx1 : DSPBAPrim/Const  primtype=const  nInputs=0  nOutputs=1  omode=boolean  otype=ufix(1)  scale=0  rndmethod=Unbiased  factor=1  satmethod=Symmetric  shift_vec=[0 1 2 -1]  value=1  inPortNames=['+'; '+';]  outPortNames=[' ']  dspbaimage=dspba_prim.jpg  text=fprintf('%s', num2str(value));  style=Optimised  visibilities=8 + 1024  floatPrecision=float32_m23  version=20120820
  Out_RFP : Outport
  wires:
  zero_idx1/1 -> GPOut/1
  GPOut/1 -> Out_RFP/1

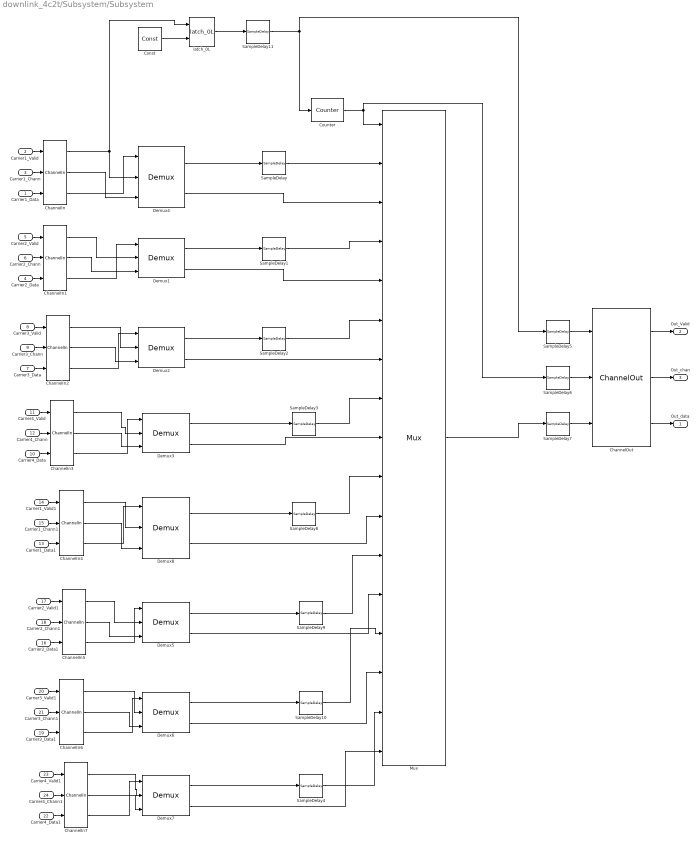
== system downlink_4c2t/Subsystem/Subsystem ==
  Carrier1_Data : Inport
  Carrier1_Valid : Inport  Port=2
  Carrier1_Chann : Inport  Port=3
  Carrier2_Data : Inport  Port=4
  Carrier2_Valid : Inport  Port=5
  Carrier2_Chann : Inport  Port=6
  Carrier3_Data : Inport  Port=7
  Carrier3_Valid : Inport  Port=8
  Carrier3_Chann : Inport  Port=9
  Carrier4_Data : Inport  Port=10
  Carrier4_Valid : Inport  Port=11
  Carrier4_Chann : Inport  Port=12
  Carrier1_Data1 : Inport  Port=13
  Carrier1_Valid1 : Inport  Port=14
  Carrier1_Chann1 : Inport  Port=15
  Carrier2_Data1 : Inport  Port=16
  Carrier2_Valid1 : Inport  Port=17
  Carrier2_Chann1 : Inport  Port=18
  Carrier3_Data1 : Inport  Port=19
  Carrier3_Valid1 : Inport  Port=20
  Carrier3_Chann1 : Inport  Port=21
  Carrier4_Data1 : Inport  Port=22
  Carrier4_Valid1 : Inport  Port=23
  Carrier4_Chann1 : Inport  Port=24
  ChannelIn{,1..7} (8 alike) : DSPBAPrim/ChannelIn  primtype=channelin  nInputs=dspba_internal_get_channel_ports(gcb)  nOutputs=dspba_internal_get_channel_ports(gcb)  omode=Inherit via internal rule  otype=sfix(16)  scale=2^-15  rndmethod=Unbiased  factor=1  satmethod=Symmetric  shift_vec=[0 1 2 -1]  value=1  inPortNames=['v'; 'c'; '0'; '1'; '2'; '3'; '4'; '5'; '6'; '7'; '8'; '9'; 'A'; 'B'; 'D'; 'E'; 'F'; 'G'; 'H'; 'I'; 'J'; 'K'; 'L'; 'M'; 'N'; 'O'; 'P'; 'Q'; 'R'; 'S'; 'T'; 'U'; 'W'; 'X'; 'Y'; 'Z']  outPortNames=['v'; 'c'; '0'; '1'; '2'; '3'; '4'; '5'; '6'; '7'; '8'; '9'; 'A'; 'B'; 'D'; 'E'; 'F'; 'G'; 'H'; 'I'; 'J'; 'K'; 'L'; 'M'; 'N'; 'O'; 'P'; 'Q'; 'R'; 'S'; 'T'; 'U'; 'W'; 'X'; 'Y'; 'Z']  dspbaimage=dspba_prim.jpg  text=fprintf('In');  style=Optimised  dataSignals=1  foldingEnabled=off  channels=1  sampleRate=200  packetBeginPresent=off  packetBeginEnabled=off  visibilities=dspba_ChannelInVis(gcb)  latencyCorrection=0  version=20141013
  ChannelOut : DSPBAPrim/ChannelOut  primtype=channelout  nInputs=dspba_internal_get_channel_ports(gcb)  nOutputs=dspba_internal_get_channel_ports(gcb)  omode=Inherit via internal rule  otype=sfix(16)  scale=2^-15  rndmethod=Unbiased  factor=1  satmethod=Symmetric  shift_vec=[0 1 2 -1]  value=1  inPortNames=['v'; 'c'; '0'; '1'; '2'; '3'; '4'; '5'; '6'; '7'; '8'; '9'; 'A'; 'B'; 'D'; 'E'; 'F'; 'G'; 'H'; 'I'; 'J'; 'K'; 'L'; 'M'; 'N'; 'O'; 'P'; 'Q'; 'R'; 'S'; 'T'; 'U'; 'W'; 'X'; 'Y'; 'Z']  outPortNames=['v'; 'c'; '0'; '1'; '2'; '3'; '4'; '5'; '6'; '7'; '8'; '9'; 'A'; 'B'; 'D'; 'E'; 'F'; 'G'; 'H'; 'I'; 'J'; 'K'; 'L'; 'M'; 'N'; 'O'; 'P'; 'Q'; 'R'; 'S'; 'T'; 'U'; 'W'; 'X'; 'Y'; 'Z']  dspbaimage=dspba_prim.jpg  text=fprintf('Out%s', AdvDSPBChannelOutDisplay(latency));  style=Optimised  dataSignals=1  foldingEnabled=off  channels=1  sampleRate=200  packetBeginPresent=off  packetBeginEnabled=off  visibilities=dspba_ChannelOutVis(gcb)  latency=0  latencyCorrection=0  version=20141013
  Const : DSPBAPrim/Const  primtype=const  nInputs=0  nOutputs=1  omode=boolean  otype=sfix(16)  scale=2^-15  rndmethod=Unbiased  factor=1  satmethod=Symmetric  shift_vec=[0 1 2 -1]  value=1  inPortNames=['+'; '+';]  outPortNames=[' ']  dspbaimage=dspba_prim.jpg  text=fprintf('%s', num2str(value));  style=Optimised  visibilities=8 + 1024  floatPrecision=float32_m23  version=20120820
  Counter : DSPBAPrim/Counter  primtype=counter  nInputs=1  nOutputs=1  omode=Inherit via internal rule  otype=ufix(16)  scale=2^-0  rndmethod=Unbiased  factor=1  satmethod=Symmetric  shift_vec=[0 1 2 -1]  value=[15 16 1]  inPortNames=[' '; ' ';]  outPortNames=[' ']  dspbaimage=dspba_prim.jpg  text=fprintf('counter\n[%d %d %d]', value(1), value(2), value(3));  style=Optimised  visibilities=8 + 1024  version=20090407
  Demux{1..8} (8 alike) : DSPBAPrim/Demux  primtype=demux  nInputs=3  nOutputs=dspba_internal_get_demux_ports(gcb)  omode=Inherit via internal rule  otype=sfix(16)  scale=2^-15  rndmethod=Unbiased  factor=1  satmethod=Symmetric  shift_vec=[0 1]  value=2  inPortNames=['q'; 'v'; 'c']  outPortNames=['c0'; 'c1']  dspbaimage=dspba_prim.jpg  text=fprintf('demux');  style=Optimised  visibilities=1536  version=20100120
  Mux : DSPBAPrim/Mux  primtype=mux  nInputs=evalAionMaskParam(gcb,'value',1)+1  nOutputs=1  omode=Inherit via internal rule  otype=sfix(16)  scale=2^-15  rndmethod=Unbiased  factor=1  satmethod=Symmetric  shift_vec=[0 1 2 -1]  value=16  inPortNames=['s'; 'd0'; 'd1'; 'd2'; 'd3'; 'd4'; 'd5'; 'd6'; 'd7'; 'd8'; 'd9';]  outPortNames=[' ']  dspbaimage=dspba_prim.jpg  text=fprintf('%s', primtype);  style=Optimised  visibilities=1032  version=20131025
  SampleDelay{,1..11} (12 alike) : DSPBAPrim/SampleDelay  primtype=sampdelay  nInputs=1  nOutputs=1  omode=Inherit via internal rule  otype=sfix(16)  scale=2^-15  rndmethod=Unbiased  factor=1  satmethod=Symmetric  shift_vec=[0 1 2 -1]  value=1  inPortNames=[' '; ' ';]  outPortNames=[' ']  dspbaimage=dspba_prim.jpg  text=dpoly(1, eye(1,value+1), 'z')  style=Optimised  visibilities=8 + 1024 + 2^17 + 2^18  flexible=off  slackgroup=0  augmented=0  version=20090407  advOptions=[]
  latch_0L : DSPBAControl/latch_0L
  Out_data : Outport
  Out_Valid : Outport  Port=2
  Out_chan : Outport  Port=3
  wires:
  Demux4/1 -> SampleDelay/1
  ChannelIn1/1 -> Demux1/2
  ChannelIn2/3 -> Demux2/1
  Carrier2_Valid/1 -> ChannelIn1/1
  Demux1/1 -> SampleDelay1/1
  Carrier3_Chann/1 -> ChannelIn2/2
  ChannelIn3/2 -> Demux3/3
  Demux2/1 -> SampleDelay2/1
  ChannelIn1/2 -> Demux1/3
  ChannelIn/3 -> Demux4/1
  Carrier2_Chann/1 -> ChannelIn1/2
  ChannelIn2/2 -> Demux2/3
  Carrier2_Data/1 -> ChannelIn1/3
  Carrier4_Data/1 -> ChannelIn3/3
  Carrier3_Data/1 -> ChannelIn2/3
  Carrier1_Valid/1 -> ChannelIn/1
  Carrier3_Valid/1 -> ChannelIn2/1
  ChannelIn3/3 -> Demux3/1
  ChannelIn3/1 -> Demux3/2
  Carrier4_Chann/1 -> ChannelIn3/2
  ChannelIn/2 -> Demux4/3
  Demux3/1 -> SampleDelay3/1
  Carrier1_Chann/1 -> ChannelIn/2
  Carrier1_Data/1 -> ChannelIn/3
  ChannelIn2/1 -> Demux2/2
  ChannelIn1/3 -> Demux1/1
  Carrier4_Valid/1 -> ChannelIn3/1
  ChannelIn/1 -> latch_0L/1, Demux4/2
  Demux8/1 -> SampleDelay8/1
  ChannelIn5/1 -> Demux5/2
  ChannelIn6/3 -> Demux6/1
  Carrier2_Valid1/1 -> ChannelIn5/1
  Demux5/1 -> SampleDelay9/1
  Carrier3_Chann1/1 -> ChannelIn6/2
  ChannelIn7/2 -> Demux7/3
  Demux6/1 -> SampleDelay10/1
  ChannelIn5/2 -> Demux5/3
  ChannelIn4/3 -> Demux8/1
  Carrier2_Chann1/1 -> ChannelIn5/2
  ChannelIn6/2 -> Demux6/3
  Carrier2_Data1/1 -> ChannelIn5/3
  Carrier4_Data1/1 -> ChannelIn7/3
  Carrier3_Data1/1 -> ChannelIn6/3
  Carrier1_Valid1/1 -> ChannelIn4/1
  Carrier3_Valid1/1 -> ChannelIn6/1
  ChannelIn7/3 -> Demux7/1
  ChannelIn7/1 -> Demux7/2
  Carrier4_Chann1/1 -> ChannelIn7/2
  ChannelIn4/2 -> Demux8/3
  Carrier1_Chann1/1 -> ChannelIn4/2
  Carrier1_Data1/1 -> ChannelIn4/3
  ChannelIn6/1 -> Demux6/2
  ChannelIn5/3 -> Demux5/1
  Carrier4_Valid1/1 -> ChannelIn7/1
  ChannelIn4/1 -> Demux8/2
  SampleDelay/1 -> Mux/2
  Demux4/2 -> Mux/3
  SampleDelay1/1 -> Mux/4
  Demux1/2 -> Mux/5
  SampleDelay2/1 -> Mux/6
  Demux2/2 -> Mux/7
  SampleDelay3/1 -> Mux/8
  Demux3/2 -> Mux/9
  SampleDelay8/1 -> Mux/10
  Demux8/2 -> Mux/11
  SampleDelay9/1 -> Mux/12
  Demux5/2 -> Mux/13
  SampleDelay10/1 -> Mux/14
  Demux6/2 -> Mux/15
  Demux7/1 -> SampleDelay4/1
  Demux7/2 -> Mux/17
  ChannelOut/3 -> Out_data/1
  ChannelOut/2 -> Out_chan/1
  ChannelOut/1 -> Out_Valid/1
  Mux/1 -> SampleDelay7/1
  SampleDelay4/1 -> Mux/16
  Counter/1 -> Mux/1, SampleDelay6/1
  Const/1 -> latch_0L/2
  latch_0L/1 -> SampleDelay11/1
  SampleDelay5/1 -> ChannelOut/1
  SampleDelay6/1 -> ChannelOut/2
  SampleDelay7/1 -> ChannelOut/3
  SampleDelay11/1 -> SampleDelay5/1, Counter/1

== system downlink_4c2t/Subsystem/Test vector Generation Unit ==
  Create Channelized  Input Data1 : DSPBAUtilities/Channelizer  data_input=DUC_LINEUP_param.inputdata_A1xC1  folding=DUC_LINEUP_param.Period_A1xC1  samples_valid=1  samples_idle=0  sample_time=1
  Create Channelized  Input Data2 : DSPBAUtilities/Channelizer  data_input=DUC_LINEUP_param.inputdata_A1xC2  folding=DUC_LINEUP_param.Period_A1xC2  samples_valid=1  samples_idle=0  sample_time=1
  Create Channelized  Input Data3 : DSPBAUtilities/Channelizer  data_input=DUC_LINEUP_param.inputdata_A1xC3  folding=DUC_LINEUP_param.Period_A1xC3  samples_valid=1  samples_idle=0  sample_time=1
  Create Channelized  Input Data4 : DSPBAUtilities/Channelizer  data_input=DUC_LINEUP_param.inputdata_A1xC4  folding=DUC_LINEUP_param.Period_A1xC4  samples_valid=1  samples_idle=0  sample_time=1
  Create Channelized  Input Data5 : DSPBAUtilities/Channelizer  data_input=DUC_LINEUP_param.inputdata_A2xC1  folding=DUC_LINEUP_param.Period_A2xC1  samples_valid=1  samples_idle=0  sample_time=1
  Create Channelized  Input Data6 : DSPBAUtilities/Channelizer  data_input=DUC_LINEUP_param.inputdata_A2xC2  folding=DUC_LINEUP_param.Period_A2xC2  samples_valid=1  samples_idle=0  sample_time=1
  Create Channelized  Input Data7 : DSPBAUtilities/Channelizer  data_input=DUC_LINEUP_param.inputdata_A2xC3  folding=DUC_LINEUP_param.Period_A2xC3  samples_valid=1  samples_idle=0  sample_time=1
  Create Channelized  Input Data8 : DSPBAUtilities/Channelizer  data_input=DUC_LINEUP_param.inputdata_A2xC4  folding=DUC_LINEUP_param.Period_A2xC4  samples_valid=1  samples_idle=0  sample_time=1
  A1xC1_Data : Outport
  A1xC1_Valid : Outport  Port=2
  A1xC1_Chan : Outport  Port=3
  A1xC2_Data : Outport  Port=4
  A1xC2_Valid : Outport  Port=5
  A1xC2_Chan : Outport  Port=6
  A1xC3_Data : Outport  Port=7
  A1xC3_Valid : Outport  Port=8
  A1xC3_Chan : Outport  Port=9
  A1xC4_Data : Outport  Port=10
  A1xC4_Valid : Outport  Port=11
  A1xC4_Chan : Outport  Port=12
  A2xC1_Data : Outport  Port=13
  A2xC1_Valid : Outport  Port=14
  A2xC1_Chan : Outport  Port=15
  A2xC2_Data : Outport  Port=16
  A2xC2_Valid : Outport  Port=17
  A2xC2_Chan : Outport  Port=18
  A2xC3_Data : Outport  Port=19
  A2xC3_Valid : Outport  Port=20
  A2xC3_Chan : Outport  Port=21
  A2xC4_Data : Outport  Port=22
  A2xC4_Valid : Outport  Port=23
  A2xC4_Chan : Outport  Port=24
  wires:
  Create Channelized  Input Data1/1 -> A1xC1_Data/1  "data signal"
  Create Channelized  Input Data2/3 -> A1xC2_Chan/1
  Create Channelized  Input Data4/1 -> A1xC4_Data/1
  Create Channelized  Input Data1/2 -> A1xC1_Valid/1  "valid signal"
  Create Channelized  Input Data3/2 -> A1xC3_Valid/1
  Create Channelized  Input Data1/3 -> A1xC1_Chan/1  "channel count signal"
  Create Channelized  Input Data4/2 -> A1xC4_Valid/1
  Create Channelized  Input Data2/1 -> A1xC2_Data/1
  Create Channelized  Input Data2/2 -> A1xC2_Valid/1
  Create Channelized  Input Data4/3 -> A1xC4_Chan/1
  Create Channelized  Input Data3/3 -> A1xC3_Chan/1
  Create Channelized  Input Data3/1 -> A1xC3_Data/1
  Create Channelized  Input Data7/1 -> A2xC3_Data/1
  Create Channelized  Input Data7/3 -> A2xC3_Chan/1
  Create Channelized  Input Data8/3 -> A2xC4_Chan/1
  Create Channelized  Input Data6/2 -> A2xC2_Valid/1
  Create Channelized  Input Data6/1 -> A2xC2_Data/1
  Create Channelized  Input Data8/2 -> A2xC4_Valid/1
  Create Channelized  Input Data5/3 -> A2xC1_Chan/1  "channel count signal"
  Create Channelized  Input Data7/2 -> A2xC3_Valid/1
  Create Channelized  Input Data5/2 -> A2xC1_Valid/1  "valid signal"
  Create Channelized  Input Data8/1 -> A2xC4_Data/1
  Create Channelized  Input Data6/3 -> A2xC2_Chan/1
  Create Channelized  Input Data5/1 -> A2xC1_Data/1  "data signal"

== system downlink_4c2t/DUT/BLIND_CFR/CFR1 ==
  In1 : Inport
  In2 : Inport  Port=2
  In3 : Inport  Port=3
  CPG gen : Subsystem
  Complex to Magnitude-Angle1 : ComplexToMagnitudeAngle  Output=Magnitude
  Complex to Magnitude-Angle2 : ComplexToMagnitudeAngle  Output=Magnitude
  Data Type Conversion2 : DataTypeConversion  OutDataTypeStr=double
  Data Type Conversion3 : DataTypeConversion  OutDataTypeStr=double
  Output2 : Scope  NumInputPorts=3
  PeakCan : Subsystem
  PulseScale : Subsystem
  Out1 : Outport
  Out2 : Outport  Port=2
  Out3 : Outport  Port=3
  wires:
  In1/1 -> PulseScale/1(v)
  In2/1 -> PulseScale/2(c)
  PeakCan/1(qv) -> Out1/1
  PeakCan/2(qc) -> Out2/1
  PeakCan/3(q) -> Out3/1
  CPG gen/3(cpg) -> Data Type Conversion2/1, PeakCan/3(d)
  CPG gen/4(sig_o) -> Data Type Conversion3/1, PeakCan/4(sig)
  CPG gen/1(qv) -> PeakCan/1(v)
  CPG gen/2(qc) -> PeakCan/2(c)
  PulseScale/1(qv) -> CPG gen/1(v)
  PulseScale/2(qc) -> CPG gen/2(c)
  PulseScale/3(Out_c) -> CPG gen/4(mag), Output2/3
  PulseScale/4(count_o) -> CPG gen/3(counter)
  Data Type Conversion2/1 -> Complex to Magnitude-Angle1/1
  Complex to Magnitude-Angle1/1 -> Output2/1
  Data Type Conversion3/1 -> Complex to Magnitude-Angle2/1
  Complex to Magnitude-Angle2/1 -> Output2/2
  In3/1 -> PulseScale/3(d)
  PulseScale/5(sig_i) -> CPG gen/5(sig_i)

== system downlink_4c2t/DUT/BLIND_CFR/CFR2 ==
  In1 : Inport
  In2 : Inport  Port=2
  In3 : Inport  Port=3
  CPG gen : Subsystem
  Complex to Magnitude-Angle1 : ComplexToMagnitudeAngle  Output=Magnitude
  Complex to Magnitude-Angle2 : ComplexToMagnitudeAngle  Output=Magnitude
  Data Type Conversion2 : DataTypeConversion  OutDataTypeStr=double
  Data Type Conversion3 : DataTypeConversion  OutDataTypeStr=double
  Output2 : Scope  NumInputPorts=3
  PeakCan : Subsystem
  PulseScale : Subsystem
  Out1 : Outport
  Out2 : Outport  Port=2
  Out3 : Outport  Port=3
  wires:
  PulseScale/5(sig_i) -> CPG gen/5(sig_i)
  In3/1 -> PulseScale/3(d)
  Complex to Magnitude-Angle2/1 -> Output2/2
  Data Type Conversion3/1 -> Complex to Magnitude-Angle2/1
  Complex to Magnitude-Angle1/1 -> Output2/1
  Data Type Conversion2/1 -> Complex to Magnitude-Angle1/1
  PulseScale/4(count_o) -> CPG gen/3(counter)
  PulseScale/3(Out_c) -> Output2/3, CPG gen/4(mag)
  PulseScale/2(qc) -> CPG gen/2(c)
  PulseScale/1(qv) -> CPG gen/1(v)
  CPG gen/2(qc) -> PeakCan/2(c)
  CPG gen/1(qv) -> PeakCan/1(v)
  CPG gen/4(sig_o) -> PeakCan/4(sig), Data Type Conversion3/1
  CPG gen/3(cpg) -> PeakCan/3(d), Data Type Conversion2/1
  PeakCan/3(q) -> Out3/1
  PeakCan/2(qc) -> Out2/1
  PeakCan/1(qv) -> Out1/1
  In2/1 -> PulseScale/2(c)
  In1/1 -> PulseScale/1(v)

== system downlink_4c2t/DUT/DPD/DPD_ANT1 ==
  note: DPD Feed forward
  valid : Inport  OutDataTypeStr=boolean  SampleTime=1
  channel : Inport  Port=2  OutDataTypeStr=uint8  SampleTime=1
  xr : Inport  Port=3  SampleTime=1
  sop : Inport  Port=4  SampleTime=1
  eop : Inport  Port=5  SampleTime=1
  Arb : Inport  Port=6  SampleTime=1
  ChannelIn1 : DSPBAPrim/ChannelIn  primtype=channelin  nInputs=dspba_internal_get_channel_ports(gcb)  nOutputs=dspba_internal_get_channel_ports(gcb)  omode=Inherit via internal rule  otype=sfix(16)  scale=2^-15  rndmethod=Unbiased  factor=1  satmethod=Symmetric  shift_vec=[0 1 2 -1]  value=4  inPortNames=['v'; 'c'; '0'; '1'; '2'; '3'; '4'; '5'; '6'; '7'; '8'; '9'; 'A'; 'B'; 'D'; 'E'; 'F'; 'G'; 'H'; 'I'; 'J'; 'K'; 'L'; 'M'; 'N'; 'O'; 'P'; 'Q'; 'R'; 'S'; 'T'; 'U'; 'W'; 'X'; 'Y'; 'Z']  outPortNames=['v'; 'c'; '0'; '1'; '2'; '3'; '4'; '5'; '6'; '7'; '8'; '9'; 'A'; 'B'; 'D'; 'E'; 'F'; 'G'; 'H'; 'I'; 'J'; 'K'; 'L'; 'M'; 'N'; 'O'; 'P'; 'Q'; 'R'; 'S'; 'T'; 'U'; 'W'; 'X'; 'Y'; 'Z']  dspbaimage=dspba_prim.jpg  text=fprintf('In');  style=Optimised  dataSignals=4  foldingEnabled=off  channels=1  sampleRate=200  packetBeginPresent=off  packetBeginEnabled=off  visibilities=dspba_ChannelInVis(gcb)  latencyCorrection=0  version=20141013
  ChannelOut1 : DSPBAPrim/ChannelOut  primtype=channelout  nInputs=dspba_internal_get_channel_ports(gcb)  nOutputs=dspba_internal_get_channel_ports(gcb)  omode=Inherit via internal rule  otype=sfix(16)  scale=2^-15  rndmethod=Unbiased  factor=1  satmethod=Symmetric  shift_vec=[0 1 2 -1]  value=3  inPortNames=['v'; 'c'; '0'; '1'; '2'; '3'; '4'; '5'; '6'; '7'; '8'; '9'; 'A'; 'B'; 'D'; 'E'; 'F'; 'G'; 'H'; 'I'; 'J'; 'K'; 'L'; 'M'; 'N'; 'O'; 'P'; 'Q'; 'R'; 'S'; 'T'; 'U'; 'W'; 'X'; 'Y'; 'Z']  outPortNames=['v'; 'c'; '0'; '1'; '2'; '3'; '4'; '5'; '6'; '7'; '8'; '9'; 'A'; 'B'; 'D'; 'E'; 'F'; 'G'; 'H'; 'I'; 'J'; 'K'; 'L'; 'M'; 'N'; 'O'; 'P'; 'Q'; 'R'; 'S'; 'T'; 'U'; 'W'; 'X'; 'Y'; 'Z']  dspbaimage=dspba_prim.jpg  text=fprintf('Out%s', AdvDSPBChannelOutDisplay(latency));  style=Optimised  dataSignals=3  foldingEnabled=off  channels=1  sampleRate=200  packetBeginPresent=off  packetBeginEnabled=off  visibilities=dspba_ChannelOutVis(gcb)  latency=41  latencyCorrection=0  version=20141013
  Convert : DSPBAPrim/Convert  primtype=convert  nInputs=1  nOutputs=1  omode=Specify via dialog  otype=sfix(16)  scale=2^-15  rndmethod=Unbiased  factor=1  satmethod=None  shift_vec=[0 1 2 -1]  value=round([0:255]/17)  inPortNames=[' '; ' ';]  outPortNames=[' '; 'c']  dspbaimage=dspba_prim.jpg  text=fprintf('convert');  style=Optimised  visibilities=8+64+256+2^17  clipdetect=off  floatPrecision=float32_m23  advOptions=[]  version=20130211
  DPD_FF : downlink_4c2t_lib/DPD_FF  LutContent=LUTS.ENTRIES  CoefWidth=16  Coeff_fractionwidth=11  DataWidth=16  fractionwidth=15  LutUpdateAddress=StartAddress1+512  LutUpdateCoeff1=StartAddress1+513  LutUpdateCoeff2=StartAddress1+514  LutUpdateCoeff3=StartAddress1+515  LutUpdateCoeff4=StartAddress1+516  LutUpdateCoeff5=StartAddress1+517  LutUpdateCoeff6=StartAddress1+518  LutUpdateCoeff7=StartAddress1+519  LutUpdateCoeff8=StartAddress1+520  DPDReadBankAddress=StartAddress1+521
  LocalThreshold : DSPBABase/LocalThreshold  margin=DUC_LINEUP_param.ClockMargin_DPD  delayRegOrRAMThresholdBits=-1  MediumDualMemThresholdBits=-1  LargeDualMemThresholdBits=-1  hardMultiplierThresholdLuts=-1  complexMultKaratsuba=off  version=0
  Mux : DSPBAPrim/Mux  primtype=mux  nInputs=evalAionMaskParam(gcb,'value',1)+1  nOutputs=1  omode=Inherit via internal rule  otype=sfix(16)  scale=2^-15  rndmethod=Unbiased  factor=1  satmethod=Symmetric  shift_vec=[0 1 2 -1]  value=2  inPortNames=['s'; 'd0'; 'd1'; 'd2'; 'd3'; 'd4'; 'd5'; 'd6'; 'd7'; 'd8'; 'd9';]  outPortNames=[' ']  dspbaimage=dspba_prim.jpg  text=fprintf('%s', primtype);  style=Optimised  visibilities=1032  version=20131025
  Predistorter Enable : DSPBAModelBus/RegField  reg_name=StartAddress1+256  reg_rwmode=Read/Write  reg_msb=0  reg_lsb=0  reg_mode=Specify via dialog  reg_type=ufix(1)  reg_scale=2^0  reg_init=enable_DPD1  reg_desc=Enable the Forward Path DPD1  reg_modal=off  reg_desc0=0  reg_desc1=0  reg_desc2=0  reg_desc3=0  reg_desc4=0  reg_desc5=0  reg_desc6=0  reg_desc7=0  reg_addr=7824  SampleTime=-1  version=20090407
  SampleDelay : DSPBAPrim/SampleDelay  primtype=sampdelay  nInputs=1  nOutputs=1  omode=Inherit via internal rule  otype=sfix(16)  scale=2^-15  rndmethod=Unbiased  factor=1  satmethod=Symmetric  shift_vec=[0 1 2 -1]  value=1  inPortNames=[' '; ' ';]  outPortNames=[' ']  dspbaimage=dspba_prim.jpg  text=dpoly(1, eye(1,value+1), 'z')  style=Optimised  visibilities=8 + 1024 + 2^17 + 2^18  flexible=off  slackgroup=0  augmented=0  version=20090407  advOptions=[]
  SynthesisInfo : DSPBAPrim/SynthesisInfo  primtype=synthinfo  nInputs=0  nOutputs=0  omode=Inherit via internal rule  otype=sfix(16)  scale=2^-15  rndmethod=Truncate  factor=1  satmethod=Symmetric  shift_vec=[0 1 2 -1]  value=99  inPortNames=[' '; ' ';]  outPortNames=[' ']  dspbaimage=dspba_prim_ctrl.jpg  text=fprintf('Style=%s', style);  style=Scheduled  visibilities=2^15+2^17+2^18+2^19  constraintInUse=on  constraintRelation=>  constraintLimit=40  bitAccurate=off  version=20150220
  Terminator1 : Terminator
  Terminator2 : Terminator
  v : Outport
  c : Outport  Port=2
  zr : Outport  Port=3
  sop_out : Outport  Port=4
  eop_out : Outport  Port=5
  wires:
  valid/1 -> ChannelIn1/1
  ChannelOut1/1 -> v/1
  channel/1 -> ChannelIn1/2
  ChannelOut1/2 -> c/1
  ChannelOut1/3 -> zr/1
  xr/1 -> ChannelIn1/3
  eop/1 -> ChannelIn1/5
  ChannelOut1/4 -> sop_out/1
  ChannelOut1/5 -> eop_out/1
  sop/1 -> ChannelIn1/4
  ChannelIn1/3 -> DPD_FF/1, Convert/1  "xr"
  ChannelIn1/5 -> ChannelOut1/5
  ChannelIn1/4 -> ChannelOut1/4
  ChannelIn1/2 -> ChannelOut1/2
  ChannelIn1/1 -> ChannelOut1/1, DPD_FF/2
  Mux/1 -> ChannelOut1/3
  Predistorter Enable/1 -> SampleDelay/1
  Arb/1 -> ChannelIn1/6
  ChannelIn1/6 -> Terminator1/1
  DPD_FF/1 -> Mux/3
  Convert/1 -> Mux/2
  DPD_FF/2 -> Terminator2/1
  SampleDelay/1 -> Mux/1
